simulink model "Direct_mapping_Model"  (R2016a)
settings: Solver=VariableStepAuto  StartTime=0.0  StopTime=2  RelTol=1e-3
undefined symbols (not defined in the file): display, Z
libraries: sm_lib x175, nesl_utility x20, simulink x10
(part 2 of 2)

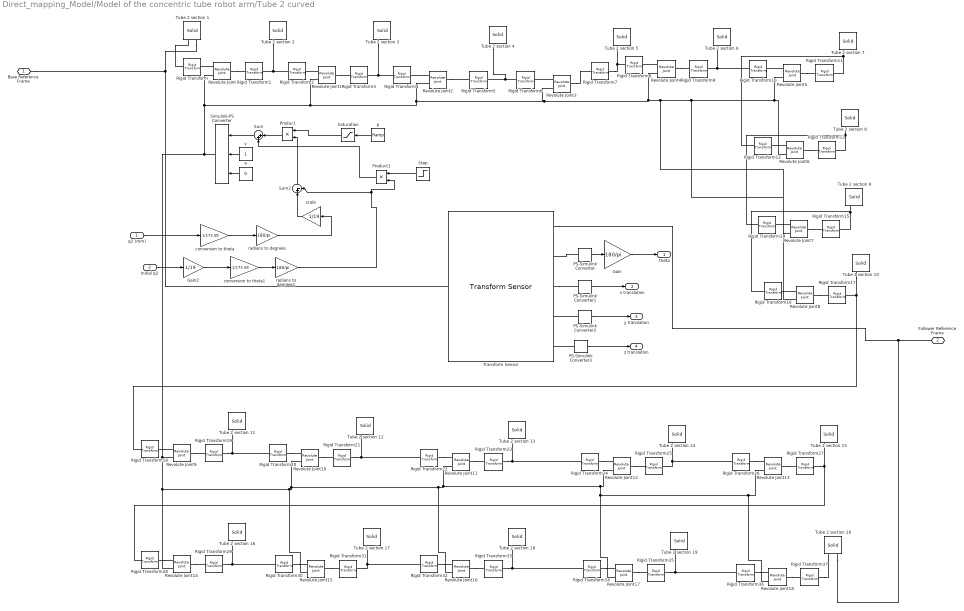
== system Direct_mapping_Model/Model of the concentric tube robot arm/Tube 2 curved ==
  q2 (mm) : Inport
  Initial q2 : Inport  Port=2
  Gain : Gain  Gain=180/pi
  Gain2 : Gain  Gain=1/19
  PS-Simulink Converter{,1..3} (4 alike) : nesl_utility/PS-Simulink Converter  PhysicalDomain=network_engine_domain  SubClassName=ps_output  LeftPortType=input  RightPortType=output  PseudoPeriodic=off  Frequencies=[]  Unit=1  AffineConversion=off
  Product : Product
  Product1 : Product
  Revolute Joint{,1..18} (19 alike) : sm_lib/Joints/Revolute Joint  SenseConstraintForce=off  SenseConstraintForceX=off  SenseConstraintForceY=off  SenseConstraintForceZ=off  SenseConstraintTorque=off  SenseConstraintTorqueX=off  SenseConstraintTorqueY=off  SenseConstraintTorqueZ=off  SenseTotalForce=off  SenseTotalForceX=off  SenseTotalForceY=off  SenseTotalForceZ=off  SenseTotalTorque=off  SenseTotalTorqueX=off  SenseTotalTorqueY=off  SenseTotalTorqueZ=off  CompositeWrenchDir=FollowerOnBase  CompositeWrenchFrame=BaseFrame  EquilibriumPosition=0  EquilibriumPositionUnits=deg  SpringStiffness=0  SpringStiffnessUnits=N*m/deg  DampingCoefficient=0  DampingCoefficientUnits=N*m/(deg/s)  TorqueActuationMode=ComputedTorque  MotionActuationMode=InputMotion  SensePosition=off  SenseVelocity=off  SenseAcceleration=off  SenseTorqueForce=off  PositionTargetSpecify=off  PositionTargetPriority=High  PositionTargetValue=0  PositionTargetValueUnits=deg  VelocityTargetSpecify=off  VelocityTargetPriority=High  VelocityTargetValue=0  VelocityTargetValueUnits=deg/s
  Rigid Transform{,2,4,6,8,10,12,14,16,18,20,22,24,26,28,30,32,34,36} (19 alike) : sm_lib/Frames and Transforms/Rigid Transform  TranslationMethod=StandardAxis  TranslationLengthUnit=mm  TranslationStandardAxis=-X  TranslationStandardOffset=173.58  TranslationCartesianOffset=[0 0 0]  TranslationROffset=0  TranslationROffsetUnits=m  TranslationZOffset=0  TranslationZOffsetUnits=m  TranslationThetaOffset=0  TranslationThetaOffsetUnits=deg  RotationMethod=StandardAxis  RotationAngleUnits=deg  RotationStandardAxis=+X  RotationAngle=90  RotationArbitraryAxis=[0 0 1]  FollAlignAxisA=+X  BaseAlignAxisA=+Y  FollAlignAxisB=+Y  BaseAlignAxisB=+Z  RotationSequenceAxes=FollowerAxes  RotationSequence=XYX  RotationSequenceAngles=[0 0 0]  RotationSequenceAnglesUnits=deg  RotationMatrix=[1 0 0; 0 1 0; 0 0 1]
  Rigid Transform{1,3,5,7,9,11,13,15,17,19,21,23,25,27,29,31,33,35,37} (19 alike) : sm_lib/Frames and Transforms/Rigid Transform  TranslationMethod=StandardAxis  TranslationLengthUnit=mm  TranslationStandardAxis=+X  TranslationStandardOffset=173.58  TranslationCartesianOffset=[0 0 0]  TranslationROffset=0  TranslationROffsetUnits=m  TranslationZOffset=0  TranslationZOffsetUnits=m  TranslationThetaOffset=0  TranslationThetaOffsetUnits=deg  RotationMethod=StandardAxis  RotationAngleUnits=deg  RotationStandardAxis=-X  RotationAngle=90  RotationArbitraryAxis=[0 0 1]  FollAlignAxisA=+X  BaseAlignAxisA=+Y  FollAlignAxisB=+Y  BaseAlignAxisB=+Z  RotationSequenceAxes=FollowerAxes  RotationSequence=XYX  RotationSequenceAngles=[0 0 0]  RotationSequenceAnglesUnits=deg  RotationMatrix=[1 0 0; 0 1 0; 0 0 1]
  Saturation : Saturate  UpperLimit=1  LowerLimit=0
  Simulink-PS Converter : nesl_utility/Simulink-PS Converter  PhysicalDomain=network_engine_domain  SubClassName=ps_input  LeftPortType=input  RightPortType=output  PseudoPeriodic=off  Frequencies=[]  NoiseDistribution=none  NoiseParameters=[]  Unit=deg  AffineConversion=off  InputFiltering=derivs  SimscapeFilterOrder=1  InputFilterTimeConstant=0.001  UdotUserProvided=2
  Step : Step  Time=0  SampleTime=0
  Sum : Sum  Inputs=|++
  Sum2 : Sum  Inputs=|+-
  Transform Sensor : sm_lib/Frames and Transforms/Transform Sensor  MeasurementFrame=Base  SenseAngle=on  SenseAxis=off  SenseAngle1=off  SenseAngle2=off  SenseAngle3=off  SenseQ=off  SenseR=off  SenseOmegaX=off  SenseOmegaY=off  SenseOmegaZ=off  SenseOmega1=off  SenseOmega2=off  SenseOmega3=off  SenseQDot=off  SenseRDot=off  SenseAlphaX=off  SenseAlphaY=off  SenseAlphaZ=off  SenseAlpha1=off  SenseAlpha2=off  SenseAlpha3=off  SenseQDDot=off  SenseRDDot=off  SenseX=on  SenseY=on  SenseZ=on  SenseRad=off  SenseAzim=off  SenseDist=off  SenseInc=off  SenseXDot=off  SenseYDot=off  SenseZDot=off  SenseRadDot=off  SenseAzimDot=off  SenseDistDot=off  SenseIncDot=off  SenseXDDot=off  SenseYDDot=off  SenseZDDot=off  SenseRadDDot=off  SenseAzimDDot=off  SenseDistDDot=off  SenseIncDDot=off
  Tube 2 section {1..20} (20 alike) : sm_lib/Body Elements/Solid  InertiaType=CalculateFromGeometry  Mass=1  MassUnits=kg  CenterOfMass=[0 0 0]  CenterOfMassUnits=m  MomentsOfInertia=[1 1 1]  MomentsOfInertiaUnits=kg*m^2  ProductsOfInertia=[0 0 0]  ProductsOfInertiaUnits=kg*m^2  DensityBased=on  Density=1000  DensityUnits=kg/(m^3)  DoExposeReferenceFrame=on  SerializedFrames=<Frames><Frame><Id>Frame1</Id><Value><Name>F1</Name><Origin><Source>GeometricFeature</Source><FeatureName>back surface</FeatureName></Origin><PrimaryAxis><DefinedDirection>-Z</DefinedDirection><Source>GeometricFeature</Source><SourceDirection>+Z</SourceDirection><FeatureName>back surface</FeatureName></PrimaryAxis><SecondaryAxis><DefinedDirection>+X</DefinedDirection><Source>ReferenceFrame</Source><SourceDirection>+X</SourceDirection><FeatureName></FeatureName></SecondaryAxis></Value></Frame><Frame><Id>Frame2</Id><Value><Name>F2</Name><Origin><Source>GeometricFeature</Source><FeatureName>front surface</FeatureName></Origin><PrimaryAxis><DefinedDirection>+Z</DefinedDirection><Source>GeometricFeature</Source><SourceDirection>+Z</SourceDirection><FeatureName>front surface</FeatureName></PrimaryAxis><SecondaryAxis><DefinedDirection>+X</DefinedDirection><Source>ReferenceFrame</Source><SourceDirection>+X</SourceDirection><FeatureName></FeatureName></SecondaryAxis></Value></Frame></Frames>  GraphicType=FromGeometry  MarkerShape=Sphere  MarkerSize=10  GraphicVisPropType=SimpleVisualProperties  GraphicDiffuseColor=[0.5 0.5 0.5]  GraphicSpecularColor=[0.5 0.5 0.5 1.0]  GraphicAmbientColor=[0.15 0.15 0.15 1.0]  GraphicEmissiveColor=[0.0 0.0 0.0 1.0]  GraphicShininess=75  GraphicOpacity=1.0  GeometryShape=GeneralSolidOfRevolution  RectangleSize=[1 1]  RectangleSizeUnits=m  BrickDimensions=[1 1 1]  BrickDimensionUnits=m  CylinderRadius=3  CylinderRadiusUnits=mm  CylinderLength=q1  CylinderLengthUnits=mm  SphereRadius=1  SphereRadiusUnits=m  EllipsoidRadii=[1 1 1]  EllipsoidRadiiUnits=m  ExtrusionCrossSection=[1 1; -1 1; -1 -1; 1 -1]  ExtrusionCrossSectionUnits=m  ExtrusionLength=1  ExtrusionLengthUnits=m  PolygonNumSides=3  PolygonOuterRadius=1  PolygonOuterRadiusUnits=m  ExtGeomFileType=STEP  ExtGeomFileUnits=m  RevolutionCrossSection=Cross_section_tube2  RevolutionCrossSectionUnits=mm  RevolutionExtent=Custom  RevolutionAngle=5  RevolutionAngleUnits=deg
  a : Constant  Value=0
  conversion to theta : Gain  Gain=1/173.58
  conversion to theta1 : Gain  Gain=1/173.58
  p : simulink/Sources/Ramp  slope=1  start=0  X0=0
  radians to degrees : Gain  Gain=180/pi
  radians to degrees1 : Gain  Gain=180/pi
  scale : Gain  Gain=1/19
  v : Constant
  Base Reference Frame : PMIOPort  Port=1  Side=Left
  Follower Reference Frame : PMIOPort  Port=2  Side=Right
  theta : Outport
  x translation : Outport  Port=2
  y translation : Outport  Port=3
  z translation : Outport  Port=4
  wires:
  a/1 -> Simulink-PS Converter/3
  v/1 -> Simulink-PS Converter/2
  p/1 -> Saturation/1
  PS-Simulink Converter/1 -> Gain/1
  Gain/1 -> theta/1
  Saturation/1 -> Product/1
  conversion to theta/1 -> radians to degrees/1
  PS-Simulink Converter1/1 -> x translation/1
  PS-Simulink Converter2/1 -> y translation/1
  PS-Simulink Converter3/1 -> z translation/1
  q2 (mm)/1 -> conversion to theta/1
  Product/1 -> Sum/1
  Sum/1 -> Simulink-PS Converter/1
  Product1/1 -> Sum/2
  Step/1 -> Product1/1
  radians to degrees1/1 -> Product1/2, Sum2/2
  conversion to theta1/1 -> radians to degrees1/1
  radians to degrees/1 -> scale/1
  Initial q2/1 -> Gain2/1
  Gain2/1 -> conversion to theta1/1
  Sum2/1 -> Product/2
  scale/1 -> Sum2/1
  connections:
  Rigid Transform/LConn1 -- Tube 2 section 1/LConn1
  Rigid Transform1/RConn1 -- Tube 2 section 2/LConn1 -- Rigid Transform2/LConn1
  Revolute Joint/LConn2 -- Revolute Joint8/LConn2 -- Revolute Joint7/LConn2 -- Revolute Joint6/LConn2 -- Revolute Joint5/LConn2 -- Revolute Joint4/LConn2 -- Revolute Joint3/LConn2 -- Revolute Joint2/LConn2 -- Revolute Joint1/LConn2 -- Revolute Joint18/LConn2 -- Revolute Joint13/LConn2 -- Revolute Joint17/LConn2 -- Revolute Joint12/LConn2 -- Revolute Joint11/LConn2 -- Revolute Joint16/LConn2 -- Revolute Joint10/LConn2 -- Revolute Joint15/LConn2 -- Revolute Joint14/LConn2 -- Revolute Joint9/LConn2 -- Simulink-PS Converter/RConn1
  Rigid Transform3/RConn1 -- Tube 2 section 3/LConn1 -- Rigid Transform4/LConn1
  Rigid Transform6/LConn1 -- Tube 2 section 4/LConn1 -- Rigid Transform5/RConn1
  Tube 2 section 5/LConn1 -- Rigid Transform7/RConn1 -- Rigid Transform8/LConn1
  Rigid Transform10/LConn1 -- Tube 2 section 6/LConn1 -- Rigid Transform9/RConn1
  Rigid Transform12/LConn1 -- Tube 2 section 7/LConn1 -- Rigid Transform11/RConn1
  Rigid Transform13/RConn1 -- Tube 2 section 8/LConn1 -- Rigid Transform14/LConn1
  Rigid Transform16/LConn1 -- Tube 2 section 9/LConn1 -- Rigid Transform15/RConn1
  Transform Sensor/RConn1 -- Tube 2 section 20/LConn2 -- Follower Reference Frame/RConn1
  Revolute Joint8/RConn1 -- Rigid Transform17/LConn1
  Revolute Joint1/RConn1 -- Rigid Transform3/LConn1
  Revolute Joint8/LConn1 -- Rigid Transform16/RConn1
  Revolute Joint2/LConn1 -- Rigid Transform4/RConn1
  Tube 2 section 10/LConn1 -- Rigid Transform18/LConn1 -- Rigid Transform17/RConn1
  Revolute Joint7/RConn1 -- Rigid Transform15/LConn1
  Revolute Joint7/LConn1 -- Rigid Transform14/RConn1
  Tube 2 section 1/LConn2 -- Base Reference Frame/RConn1 -- Transform Sensor/LConn1
  Revolute Joint3/RConn1 -- Rigid Transform7/LConn1
  PS-Simulink Converter/LConn1 -- Transform Sensor/RConn2
  Revolute Joint5/RConn1 -- Rigid Transform11/LConn1
  Revolute Joint4/RConn1 -- Rigid Transform9/LConn1
  Revolute Joint/RConn1 -- Rigid Transform1/LConn1
  Revolute Joint/LConn1 -- Rigid Transform/RConn1
  Revolute Joint1/LConn1 -- Rigid Transform2/RConn1
  Revolute Joint2/RConn1 -- Rigid Transform5/LConn1
  Revolute Joint3/LConn1 -- Rigid Transform6/RConn1
  Revolute Joint6/RConn1 -- Rigid Transform13/LConn1
  Revolute Joint4/LConn1 -- Rigid Transform8/RConn1
  Revolute Joint5/LConn1 -- Rigid Transform10/RConn1
  Revolute Joint6/LConn1 -- Rigid Transform12/RConn1
  PS-Simulink Converter3/LConn1 -- Transform Sensor/RConn5
  PS-Simulink Converter2/LConn1 -- Transform Sensor/RConn4
  Transform Sensor/RConn3 -- PS-Simulink Converter1/LConn1
  Rigid Transform18/RConn1 -- Revolute Joint9/LConn1
  Revolute Joint9/RConn1 -- Rigid Transform19/LConn1
  Rigid Transform19/RConn1 -- Rigid Transform20/LConn1 -- Tube 2 section 11/LConn1
  Rigid Transform20/RConn1 -- Revolute Joint10/LConn1
  Revolute Joint10/RConn1 -- Rigid Transform21/LConn1
  Rigid Transform21/RConn1 -- Tube 2 section 12/LConn1 -- Rigid Transform22/LConn1
  Rigid Transform22/RConn1 -- Revolute Joint11/LConn1
  Revolute Joint11/RConn1 -- Rigid Transform23/LConn1
  Rigid Transform23/RConn1 -- Rigid Transform24/LConn1 -- Tube 2 section 13/LConn1
  Rigid Transform24/RConn1 -- Revolute Joint12/LConn1
  Revolute Joint12/RConn1 -- Rigid Transform25/LConn1
  Rigid Transform25/RConn1 -- Rigid Transform26/LConn1 -- Tube 2 section 14/LConn1
  Rigid Transform26/RConn1 -- Revolute Joint13/LConn1
  Revolute Joint13/RConn1 -- Rigid Transform27/LConn1
  Rigid Transform27/RConn1 -- Rigid Transform28/LConn1 -- Tube 2 section 15/LConn1
  Rigid Transform28/RConn1 -- Revolute Joint14/LConn1
  Revolute Joint14/RConn1 -- Rigid Transform29/LConn1
  Rigid Transform29/RConn1 -- Rigid Transform30/LConn1 -- Tube 2 section 16/LConn1
  Rigid Transform30/RConn1 -- Revolute Joint15/LConn1
  Revolute Joint15/RConn1 -- Rigid Transform31/LConn1
  Rigid Transform31/RConn1 -- Rigid Transform32/LConn1 -- Tube 2 section 17/LConn1
  Rigid Transform32/RConn1 -- Revolute Joint16/LConn1
  Revolute Joint16/RConn1 -- Rigid Transform33/LConn1
  Rigid Transform33/RConn1 -- Rigid Transform34/LConn1 -- Tube 2 section 18/LConn1
  Rigid Transform34/RConn1 -- Revolute Joint17/LConn1
  Revolute Joint17/RConn1 -- Rigid Transform35/LConn1
  Rigid Transform35/RConn1 -- Rigid Transform36/LConn1 -- Tube 2 section 19/LConn1
  Rigid Transform36/RConn1 -- Revolute Joint18/LConn1
  Revolute Joint18/RConn1 -- Rigid Transform37/LConn1
  Rigid Transform37/RConn1 -- Tube 2 section 20/LConn1

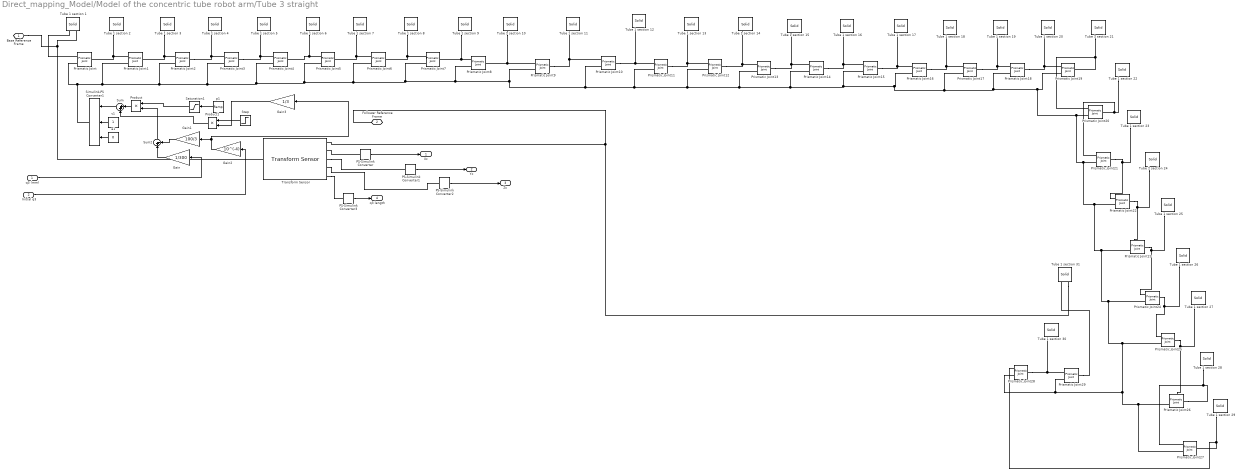
== system Direct_mapping_Model/Model of the concentric tube robot arm/Tube 3 straight ==
  q3 (mm) : Inport
  Initial q3 : Inport  Port=2
  Gain : Gain  Gain=1/300
  Gain1 : Gain  Gain=100/3
  Gain2 : Gain  Gain=10^(-4)
  Gain3 : Gain  Gain=1/3
  PS-Simulink Converter{,1..3} (4 alike) : nesl_utility/PS-Simulink Converter  PhysicalDomain=network_engine_domain  SubClassName=ps_output  LeftPortType=input  RightPortType=output  PseudoPeriodic=off  Frequencies=[]  Unit=1  AffineConversion=off
  Prismatic Joint{,1..29} (30 alike) : sm_lib/Joints/Prismatic Joint  SenseConstraintForce=off  SenseConstraintForceX=off  SenseConstraintForceY=off  SenseConstraintForceZ=off  SenseConstraintTorque=off  SenseConstraintTorqueX=off  SenseConstraintTorqueY=off  SenseConstraintTorqueZ=off  SenseTotalForce=off  SenseTotalForceX=off  SenseTotalForceY=off  SenseTotalForceZ=off  SenseTotalTorque=off  SenseTotalTorqueX=off  SenseTotalTorqueY=off  SenseTotalTorqueZ=off  CompositeWrenchDir=FollowerOnBase  CompositeWrenchFrame=BaseFrame  EquilibriumPosition=0  EquilibriumPositionUnits=m  SpringStiffness=0  SpringStiffnessUnits=N/m  DampingCoefficient=0  DampingCoefficientUnits=N/(m/s)  TorqueActuationMode=ComputedTorque  MotionActuationMode=InputMotion  SensePosition=off  SenseVelocity=off  SenseAcceleration=off  SenseTorqueForce=off  PositionTargetSpecify=off  PositionTargetPriority=High  PositionTargetValue=0  PositionTargetValueUnits=m  VelocityTargetSpecify=off  VelocityTargetPriority=High  VelocityTargetValue=0  VelocityTargetValueUnits=m/s
  Product : Product
  Product1 : Product
  Saturation1 : Saturate  UpperLimit=0.01  LowerLimit=0
  Simulink-PS Converter1 : nesl_utility/Simulink-PS Converter  PhysicalDomain=network_engine_domain  SubClassName=ps_input  LeftPortType=input  RightPortType=output  PseudoPeriodic=off  Frequencies=[]  NoiseDistribution=none  NoiseParameters=[]  Unit=m  AffineConversion=off  InputFiltering=derivs  SimscapeFilterOrder=1  InputFilterTimeConstant=0.001  UdotUserProvided=2
  Step : Step  Time=0  SampleTime=0
  Sum : Sum  Inputs=|++
  Sum2 : Sum  Inputs=|+-
  Transform Sensor : sm_lib/Frames and Transforms/Transform Sensor  MeasurementFrame=Base  SenseAngle=off  SenseAxis=off  SenseAngle1=off  SenseAngle2=off  SenseAngle3=off  SenseQ=off  SenseR=off  SenseOmegaX=off  SenseOmegaY=off  SenseOmegaZ=off  SenseOmega1=off  SenseOmega2=off  SenseOmega3=off  SenseQDot=off  SenseRDot=off  SenseAlphaX=off  SenseAlphaY=off  SenseAlphaZ=off  SenseAlpha1=off  SenseAlpha2=off  SenseAlpha3=off  SenseQDDot=off  SenseRDDot=off  SenseX=on  SenseY=on  SenseZ=on  SenseRad=off  SenseAzim=off  SenseDist=on  SenseInc=off  SenseXDot=off  SenseYDot=off  SenseZDot=off  SenseRadDot=off  SenseAzimDot=off  SenseDistDot=off  SenseIncDot=off  SenseXDDot=off  SenseYDDot=off  SenseZDDot=off  SenseRadDDot=off  SenseAzimDDot=off  SenseDistDDot=off  SenseIncDDot=off
  Tube 1 section {1..31} (31 alike) : sm_lib/Body Elements/Solid  InertiaType=CalculateFromGeometry  Mass=1  MassUnits=kg  CenterOfMass=[0 0 0]  CenterOfMassUnits=m  MomentsOfInertia=[1 1 1]  MomentsOfInertiaUnits=kg*m^2  ProductsOfInertia=[0 0 0]  ProductsOfInertiaUnits=kg*m^2  DensityBased=on  Density=0  DensityUnits=kg/(m^3)  DoExposeReferenceFrame=on  SerializedFrames=<Frames><Frame><Id>Frame1</Id><Value><Name>F1</Name><Origin><Source>GeometricFeature</Source><FeatureName>bottom surface</FeatureName></Origin><PrimaryAxis><DefinedDirection>+Z</DefinedDirection><Source>ReferenceFrame</Source><SourceDirection>+Z</SourceDirection><FeatureName></FeatureName></PrimaryAxis><SecondaryAxis><DefinedDirection>+X</DefinedDirection><Source>ReferenceFrame</Source><SourceDirection>+X</SourceDirection><FeatureName></FeatureName></SecondaryAxis></Value></Frame><Frame><Id>Frame2</Id><Value><Name>F2</Name><Origin><Source>GeometricFeature</Source><FeatureName>top surface</FeatureName></Origin><PrimaryAxis><DefinedDirection>+Z</DefinedDirection><Source>ReferenceFrame</Source><SourceDirection>+Z</SourceDirection><FeatureName></FeatureName></PrimaryAxis><SecondaryAxis><DefinedDirection>+X</DefinedDirection><Source>ReferenceFrame</Source><SourceDirection>+X</SourceDirection><FeatureName></FeatureName></SecondaryAxis></Value></Frame></Frames>  GraphicType=FromGeometry  MarkerShape=Sphere  MarkerSize=10  GraphicVisPropType=SimpleVisualProperties  GraphicDiffuseColor=[0.5 0.5 0.5]  GraphicSpecularColor=[0.5 0.5 0.5 1.0]  GraphicAmbientColor=[0.15 0.15 0.15 1.0]  GraphicEmissiveColor=[0.0 0.0 0.0 1.0]  GraphicShininess=75  GraphicOpacity=1.0  GeometryShape=Cylinder  RectangleSize=[1 1]  RectangleSizeUnits=m  BrickDimensions=[1 1 1]  BrickDimensionUnits=m  CylinderRadius=0.5  CylinderRadiusUnits=mm  CylinderLength=10  CylinderLengthUnits=mm  SphereRadius=1  SphereRadiusUnits=m  EllipsoidRadii=[1 1 1]  EllipsoidRadiiUnits=m  ExtrusionCrossSection=[1 1; -1 1; -1 -1; 1 -1]  ExtrusionCrossSectionUnits=m  ExtrusionLength=1  ExtrusionLengthUnits=m  PolygonNumSides=3  PolygonOuterRadius=1  PolygonOuterRadiusUnits=m  ExtGeomFileType=STEP  ExtGeomFileUnits=m  RevolutionCrossSection=[1 1; 1 -1; 2 -1; 2 1]  RevolutionCrossSectionUnits=m  RevolutionExtent=Full  RevolutionAngle=180  RevolutionAngleUnits=deg
  a1 : Constant  Value=0
  p1 : simulink/Sources/Ramp  slope=0.01  start=0  X0=0
  v1 : Constant
  Base Reference Frame : PMIOPort  Port=1  Side=Left
  Follower Reference Frame : PMIOPort  Port=2  Side=Right
  Xc : Outport
  Yc : Outport  Port=2
  Zc : Outport  Port=3
  q3 length : Outport  Port=4
  wires:
  a1/1 -> Simulink-PS Converter1/3
  v1/1 -> Simulink-PS Converter1/2
  p1/1 -> Saturation1/1
  Saturation1/1 -> Product/1
  PS-Simulink Converter/1 -> Xc/1
  PS-Simulink Converter1/1 -> Yc/1
  PS-Simulink Converter2/1 -> Zc/1
  PS-Simulink Converter3/1 -> q3 length/1
  Product/1 -> Sum/1
  Sum/1 -> Simulink-PS Converter1/1
  q3 (mm)/1 -> Gain/1
  Step/1 -> Product1/1
  Product1/1 -> Sum/2
  Sum2/1 -> Product/2
  Gain/1 -> Sum2/1
  Initial q3/1 -> Gain2/1
  Gain1/1 -> Sum2/2
  Gain2/1 -> Gain3/1, Gain1/1
  Gain3/1 -> Product1/2
  connections:
  Simulink-PS Converter1/RConn1 -- Prismatic Joint/LConn2 -- Prismatic Joint29/LConn2 -- Prismatic Joint28/LConn2 -- Prismatic Joint27/LConn2 -- Prismatic Joint26/LConn2 -- Prismatic Joint25/LConn2 -- Prismatic Joint24/LConn2 -- Prismatic Joint23/LConn2 -- Prismatic Joint22/LConn2 -- Prismatic Joint21/LConn2 -- Prismatic Joint20/LConn2 -- Prismatic Joint19/LConn2 -- Prismatic Joint18/LConn2 -- Prismatic Joint17/LConn2 -- Prismatic Joint16/LConn2 -- Prismatic Joint15/LConn2 -- Prismatic Joint14/LConn2 -- Prismatic Joint13/LConn2 -- Prismatic Joint12/LConn2 -- Prismatic Joint11/LConn2 -- Prismatic Joint10/LConn2 -- Prismatic Joint9/LConn2 -- Prismatic Joint8/LConn2 -- Prismatic Joint7/LConn2 -- Prismatic Joint6/LConn2 -- Prismatic Joint5/LConn2 -- Prismatic Joint4/LConn2 -- Prismatic Joint3/LConn2 -- Prismatic Joint2/LConn2 -- Prismatic Joint1/LConn2
  Tube 1 section 1/LConn1 -- Prismatic Joint/LConn1
  Prismatic Joint1/LConn1 -- Prismatic Joint/RConn1 -- Tube 1 section 2/LConn1
  Prismatic Joint2/LConn1 -- Prismatic Joint1/RConn1 -- Tube 1 section 3/LConn1
  Prismatic Joint3/LConn1 -- Tube 1 section 4/LConn1 -- Prismatic Joint2/RConn1
  Prismatic Joint4/LConn1 -- Tube 1 section 5/LConn1 -- Prismatic Joint3/RConn1
  Prismatic Joint4/RConn1 -- Tube 1 section 6/LConn1 -- Prismatic Joint5/LConn1
  Prismatic Joint6/LConn1 -- Prismatic Joint5/RConn1 -- Tube 1 section 7/LConn1
  Prismatic Joint7/LConn1 -- Prismatic Joint6/RConn1 -- Tube 1 section 8/LConn1
  Prismatic Joint8/LConn1 -- Prismatic Joint7/RConn1 -- Tube 1 section 9/LConn1
  Prismatic Joint9/LConn1 -- Tube 1 section 10/LConn1 -- Prismatic Joint8/RConn1
  Prismatic Joint9/RConn1 -- Prismatic Joint10/LConn1 -- Tube 1 section 11/LConn1
  Transform Sensor/LConn1 -- Base Reference Frame/RConn1 -- Tube 1 section 1/LConn2
  Follower Reference Frame/RConn1 -- Tube 1 section 31/LConn2 -- Transform Sensor/RConn1
  PS-Simulink Converter/LConn1 -- Transform Sensor/RConn2
  Transform Sensor/RConn3 -- PS-Simulink Converter1/LConn1
  Transform Sensor/RConn4 -- PS-Simulink Converter2/LConn1
  Prismatic Joint10/RConn1 -- Tube 1 section 12/LConn1 -- Prismatic Joint11/LConn1
  Prismatic Joint11/RConn1 -- Prismatic Joint12/LConn1 -- Tube 1 section 13/LConn1
  Prismatic Joint12/RConn1 -- Prismatic Joint13/LConn1 -- Tube 1 section 14/LConn1
  Prismatic Joint13/RConn1 -- Prismatic Joint14/LConn1 -- Tube 1 section 15/LConn1
  Prismatic Joint14/RConn1 -- Prismatic Joint15/LConn1 -- Tube 1 section 16/LConn1
  Prismatic Joint15/RConn1 -- Prismatic Joint16/LConn1 -- Tube 1 section 17/LConn1
  Prismatic Joint16/RConn1 -- Prismatic Joint17/LConn1 -- Tube 1 section 18/LConn1
  Prismatic Joint17/RConn1 -- Prismatic Joint18/LConn1 -- Tube 1 section 19/LConn1
  Prismatic Joint18/RConn1 -- Prismatic Joint19/LConn1 -- Tube 1 section 20/LConn1
  Tube 1 section 21/LConn1 -- Prismatic Joint20/LConn1 -- Prismatic Joint19/RConn1
  Tube 1 section 22/LConn1 -- Prismatic Joint21/LConn1 -- Prismatic Joint20/RConn1
  Prismatic Joint21/RConn1 -- Tube 1 section 23/LConn1 -- Prismatic Joint22/LConn1
  Prismatic Joint22/RConn1 -- Tube 1 section 24/LConn1 -- Prismatic Joint23/LConn1
  Prismatic Joint23/RConn1 -- Tube 1 section 25/LConn1 -- Prismatic Joint24/LConn1
  Prismatic Joint24/RConn1 -- Tube 1 section 26/LConn1 -- Prismatic Joint25/LConn1
  Prismatic Joint25/RConn1 -- Tube 1 section 27/LConn1 -- Prismatic Joint26/LConn1
  Prismatic Joint26/RConn1 -- Prismatic Joint27/LConn1 -- Tube 1 section 28/LConn1
  Tube 1 section 29/LConn1 -- Prismatic Joint28/LConn1 -- Prismatic Joint27/RConn1
  Prismatic Joint28/RConn1 -- Prismatic Joint29/LConn1 -- Tube 1 section 30/LConn1
  Prismatic Joint29/RConn1 -- Tube 1 section 31/LConn1
  Transform Sensor/RConn5 -- PS-Simulink Converter3/LConn1

== matlab function Direct_mapping_Model/Inverse Kinematics Code/Inverse_Kinematics_Code ==
  data: X input; q1 output; Y input; Z input; P input; Roll input; q2 output; q3 output; q4 output; q5 output; q6 output; q7 output; d input
function [q1,q2,q3,q4,q5,q6,q7] = fcn(X,Y,Z,P,Roll,d)
%This Code is the algorithm to solve the inverse kinematics.
%There are 3 cases, the general case, the minimum pitch and the maximum
%pitch. This code will give motor commands that will satisfy position the
%most it can before saturation of tube elongation

%Special Functions
coder.extrinsic('clc')
coder.extrinsic('display')
clc

%Algorithm Constants:
r = 173.58; %curved pipe curvature
q1max = 77.25; q2max = 82.5; q3max = 97.5;

R = sqrt(X^2+Y^2); %Radial Distance

% General Rotation motors Solutions
q7 = Roll;
q6 = atan2(Y,X) + (pi/2); %Offset angle from origin = 90deg
q5 = 0; %Inactive
% Forceps
q4 = d;


%******ALGORITHM TO FIND SOLUTIONS TO THE TOOL POINT POSITION***********%

%*********1 Tube Straight Solution***********%
if R == 0
    q2 = 0;
    q3 = 0.5*Z;
    q1 = 0.5*Z;
    if (q1>q1max)
        q1 = q1max; q3 = Z-q1;
    end
    display('Notice: Used 1 tube solution');
else
    %************************GENERAL CASE SOLUTION***********************%
    %Tube Elongation motors:
    q2 = r*atan2(R,(Y/tan(P)));
    %q2 = r*atan2(sqrt(tan(P)^2 + tan(Y)^2 ),1); both pitch and yaw
    C = cos(q2/r);
    S = sin(q2/r);
    q3 = ( R - r*sqrt(C^2-2*C+1) ) / S;
    q1 = Z - q3*C - r*S;
    
    %Check solution
    if (willClip(q1,q2,q3)==false)
        display('Notice: Used General 3 tube Solution');
        %Correct
    else
    %********TRY 2 TUBE SOLUTIONS*************%
        if (abs(P)>(q2max/r))
    %******************EXPECTED MAXIMUM CURVATURE SOLUTION***************%
            if (R >= (r*(1 - cos(q2max / r)))) 
					q2 = q2max;
					q3 = (R - r*(1 - cos(q2max / r)) / (sin(q2max / r)));
					q1 = Z - q3*cos(q2max / r) - r*sin(q2max / r);
                    display('Notice: Used Maximum Curvature 2 Tube Solution');
			else 
					q3 = 0;
					q2 = r* acos(1 - R / r);
					q1 = Z - r*sin(q2 / r);
                    display('Notice: Used Maximum Curvature 2 Tube Solution');
            end
        else
    %******************EXPECTED MINIMUM CURVATURE SOLUTION***************%
				a = ((R - r)*(R - r) / (Z*Z)) + 1;
				b = 2 * (R - r)*r / (Z*Z);
				c = r*r / (Z*Z) - 1;
				cosine_solution1 = (-b + sqrt(b*b - 4 * a*c)) / (2 * a);
				cosine_solution2 = (-b - sqrt(b*b - 4 * a*c)) / (2 * a);
				%%Pick solution
				if (cosine_solution1<1 || cosine_solution1>0) 
					q2 = r*acos(cosine_solution1);
					q3 = (R - r*(1 - cosine_solution1)) / sqrt(1 - cosine_solution1*cosine_solution1);
					q1 = 0;
                elseif (cosine_solution2<1 || cosine_solution2>0) 
					q2 = r*acos(cosine_solution2);
					q3 = (R - r*(1 - cosine_solution2)) / sqrt(1 - cosine_solution2*cosine_solution2);
					q1 = 0;
                end

				if (q3 > q3max) 
					a = ((r*r)/(q3max*q3max)) + 1;
					b = 2 * (R - r)*r / (q3max*q3max);
					c = (((R-r)*(R-r)) / (q3max*q3max)) - 1;
					cosine_solution1 = (-b + sqrt(b*b - 4 * a*c)) / (2 * a);
					cosine_solution2 = (-b - sqrt(b*b - 4 * a*c)) / (2 * a);
					if (cosine_solution1<1 || cosine_solution1>0)
						q2 = r*acos(cosine_solution1);
						q3 = q3max;
						q1 = Z - q3max*cosine_solution1 - r*sqrt(1-(cosine_solution1*cosine_solution1));
                    elseif (cosine_solution2<1 || cosine_solution2>0) 
						q2 = r*acos(cosine_solution2);
						q3 = q3max;
						q1 = Z - q3max*cosine_solution2 - r*sqrt(1 - (cosine_solution2*cosine_solution2));
					else 
						 display('Error: no solution found at all this error means that the selected position is invalid');
                    end
                    
                end
        end
    end

    %********Check Workspace Boundaries********%
        Z_max = q1max + q3max;
        Z1 = r*sin(q2max / r); 
        Z2 = Z1 + q3max * cos(q2max / r); 
        Z3 = Z2 + q1max; 
        R_limit1 = r*(1 - cos(q2max / r)); 
        R_limit2 = R_limit1 + q3max*sin(q2max / r); 
        M = (R_limit2 - R_limit1) / (Z2 - Z1); 
        c = R_limit1 - M*Z1; 
        M_m = (R_limit2) / (Z3 - Z_max); 
        c_m = R_limit2 - M*Z3;
    if (Z < 0) 
 
    elseif (Z <= Z1)
		R_limit = r-sqrt(r^2-Z^2);
		if (R > R_limit) 
            display('ERROR: Desired position is outside the boundary');
        end
    elseif (Z <= Z2)  
		R_limit = M*Z + c;
		if (R > R_limit) 
             display('ERROR: Desired position is outside the boundary');
        end
    elseif (Z < Z3)
		R_limit = R_limit2;
		if (R > R_limit) 
             display('ERROR: Desired position is outside the boundary');
        end
    elseif (Z <= Z3) 
		R_limit = M_m*Z + c_m;
		if (R >= R_limit2) 
             display('ERROR: Desired position is outside the boundary');
        elseif (R <= R_limit) 
             display('ERROR: Desired position is outside the boundary');
        end
    end
    
end

end

function [T] = willClip(q1a,q2a,q3a)
q1max = 77.25; q2max = 82.5; q3max = 97.5;
    if (q1a < 0)||(q2a < 0)||(q3a < 0)
        T = true;
    elseif (q1a > q1max)||(q2a > q2max)||(q3a > q3max)
        T = true;
    else
        T = false;
    end
end
